simulink model "fuzzy_sim"  (Simulink 8.5)
settings: Solver=ode45  StartTime=0.0  StopTime=5.5  MaxStep=0.001  RelTol=1e-3
libraries: fuzblock x1, simulink x1
settings Model: Creator=Windows.10  LastModifiedBy=Windows.10
settings DataIOCC: SignalLoggingSaveFormat=Dataset
settings OptimizationCC: ExpressionDepthLimit=128
settings DebuggingCC: UnderspecifiedInitializationDetection=Simplified  MergeDetectMultiDrivingBlocksExec=error  FcnCallInpInsideContextMsg=EnableAllAsError  StateNameClashWarn=none
settings GRTTargetCC: CombineOutputUpdateFcns=on  GRTInterface=off
settings ConfigurationSet: Description=SimMechanics 2G

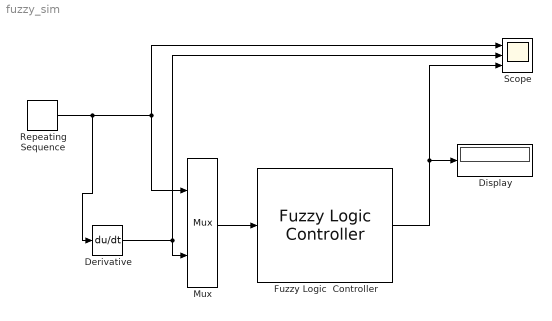
== system fuzzy_sim ==
  Derivative : Derivative
  Display : Display
  Fuzzy Logic  Controller : fuzblock/Fuzzy Logic  Controller  fis='T7km3.fis'
  Mux : Mux  Inputs=2
  Repeating Sequence : simulink/Sources/Repeating Sequence  rep_seq_t="[0 0.1 0.2 0.3 0.4 0.5  0.6 0.7 ]*10"  rep_seq_y=[0 1 1 0 -1 -1 0 0 ]
  Scope : Scope  NumInputPorts=3
      settings: YMin=-1.1~-1.11~5  YMax=1.1~1.1~6.75
  wires:
  Mux/1 -> Fuzzy Logic  Controller/1
  Fuzzy Logic  Controller/1 -> Scope/3, Display/1
  Repeating Sequence/1 -> Mux/1, Scope/1, Derivative/1
  Derivative/1 -> Scope/2, Mux/2
